simulink model "nuri3s_PDG_uncertain1"  (R2024b)
settings: Solver=VariableStepAuto  StartTime=0.0  StopTime=10  RelTol=1e-3
undefined symbols (not defined in the file): robot, timepoints, waypoints
libraries: robotmaniplib x2, robotcorelib x1
settings Model: Creator=user  LastModifiedBy=변재형

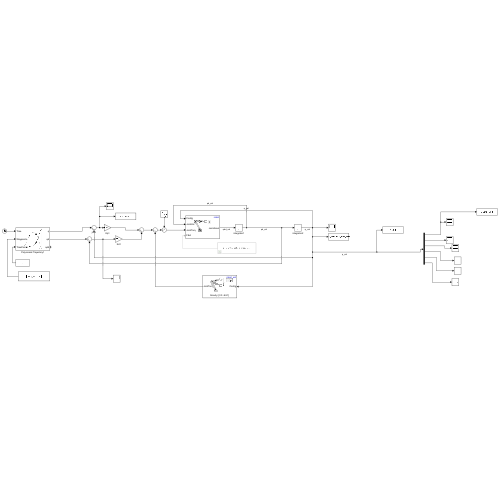
[thumbnail: Simulink's stored preview of the top-level diagram]
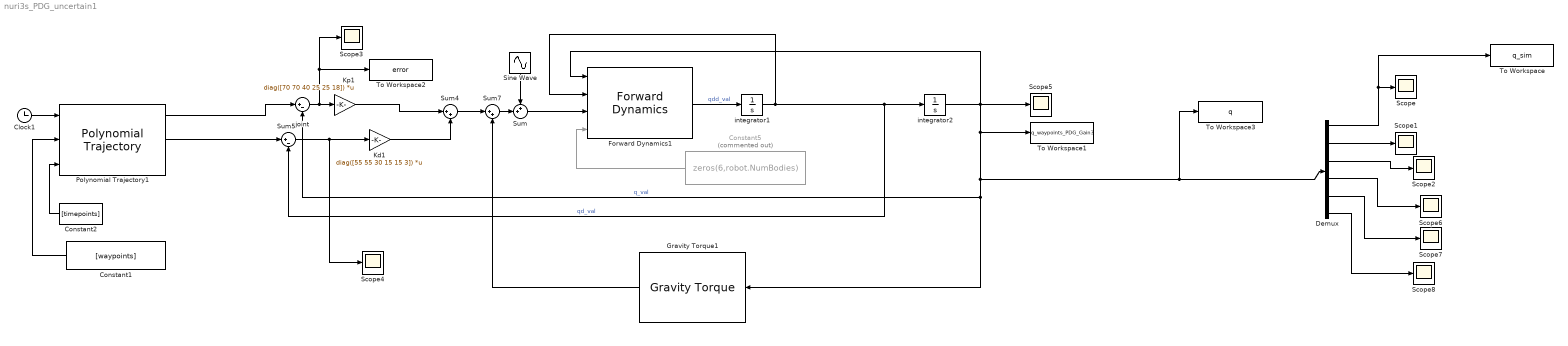
== system nuri3s_PDG_uncertain1 ==
  Clock1 : Clock
      settings: Decimation=5
  Constant1 : Constant  Value=[waypoints]
  Constant2 : Constant  Value=[timepoints]
  Constant5 : Constant  Commented=on  Value=zeros(6,robot.NumBodies)
  Demux : Demux  Outputs=6
  Forward Dynamics1 : robotmaniplib/Forward Dynamics  RigidBodyTree=robot  SimulateUsing=Interpreted execution
  Gravity Torque1 : robotmaniplib/Gravity Torque  RigidBodyTree=robot_est  SimulateUsing=Interpreted execution
  Kd1 : Gain  Gain=diag([55 55 30 15 15 3])  Multiplication=Matrix(K*u)
  Kp1 : Gain  Gain=diag([70 70 40 25 25 18])  Multiplication=Matrix(K*u)
  Polynomial Trajectory1 : robotcorelib/Polynomial Trajectory  WaypointSource=External  Waypoints=[ 0, 2, 1, 5, 0; -1, 3, 1, 4, 4 ]  TimePoints=[ 0, 1, 2, 3, 4 ]  TimeInterval=[ 1, 4 ]  Method=Quintic Polynomial  ParameterSource=Internal  VelocityBoundaryCondition=zeros( 6, 100 )  AccelerationBoundaryCondition=zeros( 6, 100 )  SimulateUsing=Interpreted execution
  Scope{,1..8} (9 alike) : Scope
  Sine Wave : Sin  Amplitude=0.1  Frequency=10  SampleTime=0
  Sum : Sum  Inputs=++|
  Sum4 : Sum  Inputs=|++
  Sum5 : Sum  Inputs=|+-
  Sum7 : Sum  Inputs=|++
  To Workspace : ToWorkspace  VariableName=q_sim  SampleTime=-1
  To Workspace1 : ToWorkspace  VariableName=q_waypoints_PDG_Gain3  SampleTime=-1
  To Workspace2 : ToWorkspace  VariableName=error  SaveFormat=Structure With Time  SampleTime=-1
  To Workspace3 : ToWorkspace  VariableName=q  SaveFormat=Structure With Time  SampleTime=-1
  integrator1 : Integrator  InitialCondition=[0 0 -1.57 0 -1.57 0]
  integrator2 : Integrator  InitialCondition=[0 0 -1.57 0 -1.57 0]
  joint : Sum  Inputs=|+-
  wires:
  Gravity Torque1/1 -> Sum7/2
  joint/1 -> Scope3/1, To Workspace2/1, Kp1/1
  Sum4/1 -> Sum7/1
  integrator2/1 -> To Workspace1/1, To Workspace3/1, Demux/1, joint/2, Gravity Torque1/1, Scope5/1, Forward Dynamics1/1  "q_val"
  integrator1/1 -> integrator2/1, Sum5/2, Forward Dynamics1/2  "qd_val"
  Forward Dynamics1/1 -> integrator1/1  "qdd_val"
  Constant5/1 -> Forward Dynamics1/4
  Sum5/1 -> Kd1/1, Scope4/1
  Kd1/1 -> Sum4/2
  Kp1/1 -> Sum4/1
  Polynomial Trajectory1/2 -> Sum5/1
  Polynomial Trajectory1/1 -> joint/1
  Constant1/1 -> Polynomial Trajectory1/2
  Constant2/1 -> Polynomial Trajectory1/3
  Clock1/1 -> Polynomial Trajectory1/1
  Demux/1 -> To Workspace/1, Scope/1
  Demux/2 -> Scope1/1
  Demux/3 -> Scope2/1
  Demux/4 -> Scope6/1
  Demux/5 -> Scope7/1
  Demux/6 -> Scope8/1
  Sum7/1 -> Sum/2
  Sum/1 -> Forward Dynamics1/3
  Sine Wave/1 -> Sum/1
